simulink model "balancingControllerWithNonLinearImpedances"  (R2012b)
settings: Solver=FixedStepDiscrete  StartTime=0.0  StopTime=inf  FixedStep=Ts  RelTol=1e-3
InitFcn:
  | initBalancingControllerWithNonLinearImpedances;
values from neighbouring files (symbols this model uses):
  damping = [dampTorso,dampArms,dampArms,dampLegs,dampLegs]*0    [initBalancingControllerWithNonLinearImpedances.m]
  gainsIDMomentum = [ 0     1   1 ]    [initBalancingControllerWithNonLinearImpedances.m]
  gainsPCOM = diag([80  80 80])    [initBalancingControllerWithNonLinearImpedances.m]
  impedances = [impTorso(1,:),impArms(1,:),impArms(1,:),impLegs(1,:),impLegs(1,:)]    [initBalancingControllerWithNonLinearImpedances.m]    (also in initBalancingController_QP.m)
  impedencesSat = [100   100    2000]    [initBalancingControllerWithNonLinearImpedances.m]    (also in initBalancingController_QP.m = [100   100    1000])
  increasingRatesGainsPCOM = [ 0     0    ]    [initBalancingControllerWithNonLinearImpedances.m]
  increasingRatesImp = [impTorso(2,:),impArms(2,:),impArms(2,:),impLegs(2,:),impLegs(2,:)]    [initBalancingControllerWithNonLinearImpedances.m]    (also in initBalancingController_QP.m)
  maxCoMx_y = [ 0.1    0.05 ]    [initBalancingControllerWithNonLinearImpedances.m]
  minCoMx_y = [-0.1   -0.25 ]    [initBalancingControllerWithNonLinearImpedances.m]
  referenceParams = [0.0 0.0]    [initBalancingControllerWithNonLinearImpedances.m]    (also in initBalancingController_QP.m = [0.04 0.25])
  satGainsPCOM = 300    [initBalancingControllerWithNonLinearImpedances.m]
undefined symbols (not defined in the file or in its folder): DiscIntNeverNeededParam
libraries: WBCLibrary x22
settings Model: Creator=daniele  LastModifiedBy=daniele
settings DataIOCC: SignalLoggingSaveFormat=ModelDataLogs
settings DebuggingCC: MultiTaskDSMMsg=warning  MultiTaskCondExecSysMsg=none  FcnCallInpInsideContextMsg=EnableAllAsWarning  StrictBusMsg=None
settings SFSimCC: SimParseCustomCode=off
settings RTWCC: IncludeERTFirstTime=on
settings CodeAppCC: CustomSymbolStrType=$N$R$M_T  InternalIdentifier=Shortened
settings GRTTargetCC: CodeReplacementLibrary=None  CombineOutputUpdateFcns=off  CPPClassGenCompliant=on  GRTInterface=on

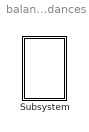
== system balancingControllerWithNonLinearImpedances ==
  Subsystem : Subsystem  mask{robotName='iCubGenova01', Ts=0.01, localName='dynamicBalancing'}
      mask prompts: robotName "robot name"; localName "module name"

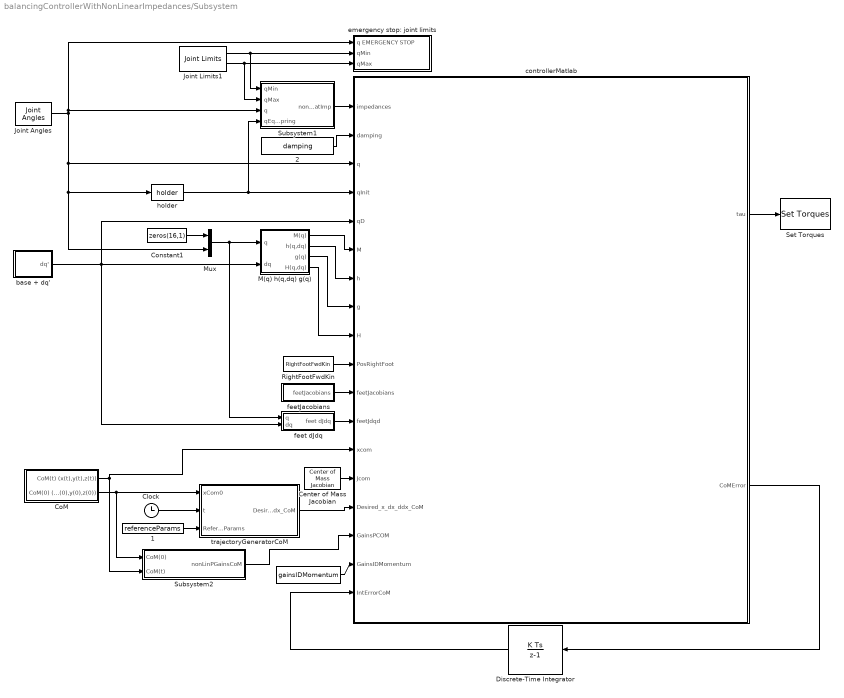
== system balancingControllerWithNonLinearImpedances/Subsystem ==
  " " : Constant  Value=gainsIDMomentum
  " 1" : Constant  Value=referenceParams
  " 2" : Constant  Value=damping
  Center of Mass Jacobian : WBCLibrary/wholeBodyModel/Jacobians/Center of Mass Jacobian  robotName=robotName  localName=localName
  Clock : Clock
  "CoM " : Subsystem
  Constant1 : Constant  Value=zeros(16,1)
  Discrete-Time Integrator : DiscreteIntegrator  InitialCondition=[0 0 0]  SampleTime=Ts  ICPrevOutput=DiscIntNeverNeededParam  ICPrevScaledInput=DiscIntNeverNeededParam
  Joint Angles : WBCLibrary/wholeBodyStates/Joint Angles  robotName=robotName  localName=localName
  Joint Limits1 : WBCLibrary/wholeBodyModel/Joint Limits  robotName=robotName  localName=localName
  M(q) h(q,dq) g(q) : Subsystem
  Mux : Mux  Inputs=2
  RightFootFwdKin : WBCLibrary/wholeBodyModel/Forward Kinematics/RightFootFwdKin  robotName=robotName  localName=localName
  Set Torques : WBCLibrary/wholeBodyActuators/Set Torques  val=6  robotName=robotName  localName=localName
  Subsystem1 : Subsystem
  Subsystem2 : Subsystem
  base + dq' : Subsystem
  controllerMatlab : MATLAB Function  TreatAsAtomicUnit=on
  emergency stop: joint limits : Subsystem
  feet dJdq : Subsystem
  feetJacobians : Subsystem
  "holder " : WBCLibrary/Utilities/holder 
  trajectoryGeneratorCoM : MATLAB Function  TreatAsAtomicUnit=on
  wires:
  trajectoryGeneratorCoM/1(Desired_x_dx_ddx_CoM) -> controllerMatlab/15(Desired_x_dx_ddx_CoM)
  Clock/1 -> trajectoryGeneratorCoM/2(t)
  "CoM "/2(CoM(0) (x(0),y(0),z(0))) -> Subsystem2/1(CoM(0)), trajectoryGeneratorCoM/1(xCom0)
  RightFootFwdKin/1 -> controllerMatlab/10(PosRightFoot)
  Discrete-Time Integrator/1 -> controllerMatlab/18(IntErrorCoM)
  Mux/1 -> M(q) h(q,dq) g(q)/1(q), feet dJdq/1(q)
  base + dq'/1(dq') -> controllerMatlab/5(qD), feet dJdq/2(dq), M(q) h(q,dq) g(q)/2(dq)
  M(q) h(q,dq) g(q)/1(M(q)) -> controllerMatlab/6(M)
  M(q) h(q,dq) g(q)/2(h(q,dq)) -> controllerMatlab/7(h)
  M(q) h(q,dq) g(q)/3(g(q)) -> controllerMatlab/8(g)
  "CoM "/1(CoM(t) (x(t),y(t),z(t))) -> Subsystem2/2(CoM(t)), controllerMatlab/13(xcom)
  M(q) h(q,dq) g(q)/4(H(q,dq)) -> controllerMatlab/9(H)
  Center of Mass Jacobian/1 -> controllerMatlab/14(Jcom)
  feetJacobians/1(feetJacobians) -> controllerMatlab/11(feetJacobians)
  feet dJdq/1(feet dJdq) -> controllerMatlab/12(feetJdqd)
  controllerMatlab/1(tau) -> Set Torques/1
  "holder "/1 -> Subsystem1/4(qEquSpring), controllerMatlab/4(qInit)
  Constant1/1 -> Mux/1
  Joint Limits1/1 -> Subsystem1/1(qMin), emergency stop: joint limits/2(qMin)
  Joint Limits1/2 -> Subsystem1/2(qMax), emergency stop: joint limits/3(qMax)
  Joint Angles/1 -> emergency stop: joint limits/1(q EMERGENCY STOP), Subsystem1/3(q), Mux/2, "holder "/1, controllerMatlab/3(q)
  Subsystem1/1(nonLinSatImp) -> controllerMatlab/1(impedances)
  controllerMatlab/2(CoMError) -> Discrete-Time Integrator/1
  " 1"/1 -> trajectoryGeneratorCoM/3(ReferenceParams)
  " "/1 -> controllerMatlab/17(GainsIDMomentum)
  Subsystem2/1(nonLinPGainsCoM) -> controllerMatlab/16(GainsPCOM)
  " 2"/1 -> controllerMatlab/2(damping)

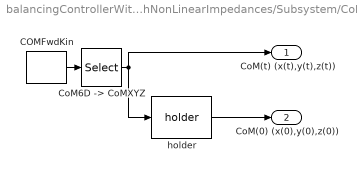
== system balancingControllerWithNonLinearImpedances/Subsystem/CoM  ==
  "COMFwdKin " : WBCLibrary/wholeBodyModel/Forward Kinematics/COMFwdKin   robotName=robotName  localName=localName
  "CoM6D -> CoMXYZ" : Selector  InputPortWidth=7  IndexOptions=Index vector (dialog)  Indices=[1 2 3]  OutputSizes=1
  "holder " : WBCLibrary/Utilities/holder 
  CoM(t) (x(t),y(t),z(t)) : Outport
  CoM(0) (x(0),y(0),z(0)) : Outport  Port=2
  wires:
  "COMFwdKin "/1 -> "CoM6D -> CoMXYZ"/1
  "CoM6D -> CoMXYZ"/1 -> "holder "/1, CoM(t) (x(t),y(t),z(t))/1
  "holder "/1 -> CoM(0) (x(0),y(0),z(0))/1

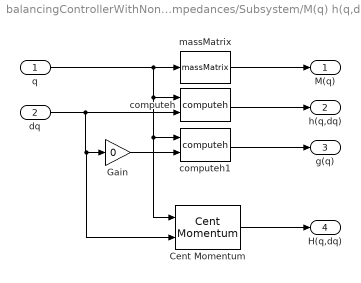
== system balancingControllerWithNonLinearImpedances/Subsystem/M(q) h(q,dq) g(q) ==
  q : Inport
  dq : Inport  Port=2
  Cent Momentum : WBCLibrary/wholeBodyModel/Dynamics/Cent Momentum  robotName=robotName  localName=localName
  Gain : Gain  Gain=0
  computeh : WBCLibrary/wholeBodyModel/Dynamics/computeh  val=7  robotname=robotName  localname=localName
  computeh1 : WBCLibrary/wholeBodyModel/Dynamics/computeh  val=7  robotname=robotName  localname=localName
  massMatrix : WBCLibrary/wholeBodyModel/Dynamics/massMatrix  val=8  robotname=robotName  localname=localName
  M(q) : Outport
  h(q,dq) : Outport  Port=2
  g(q) : Outport  Port=3
  H(q,dq) : Outport  Port=4
  wires:
  Gain/1 -> computeh1/2
  computeh1/1 -> g(q)/1
  computeh/1 -> h(q,dq)/1
  massMatrix/1 -> M(q)/1
  q/1 -> Cent Momentum/1, computeh1/1, computeh/1, massMatrix/1
  dq/1 -> Cent Momentum/2, Gain/1, computeh/2
  Cent Momentum/1 -> H(q,dq)/1

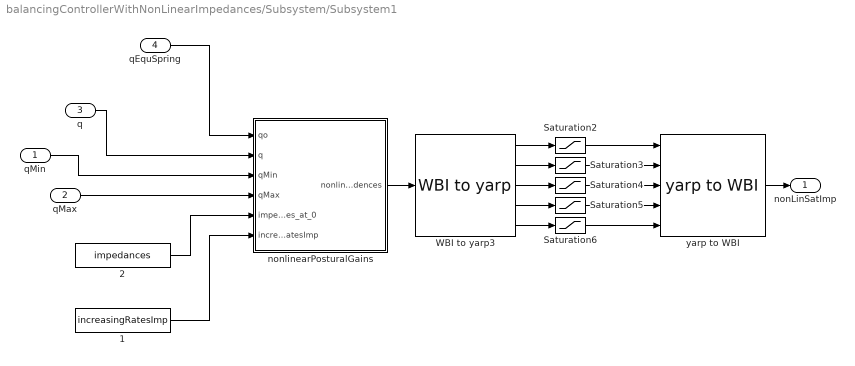
== system balancingControllerWithNonLinearImpedances/Subsystem/Subsystem1 ==
  qMin : Inport
  qMax : Inport  Port=2
  q : Inport  Port=3
  qEquSpring : Inport  Port=4
  " 1" : Constant  Value=increasingRatesImp
  " 2" : Constant  Value=impedances
  Saturation2 : Saturate  UpperLimit=impedencesSat(1)  LowerLimit=0  SampleTime=Ts
  Saturation3 : Saturate  UpperLimit=impedencesSat(2)  LowerLimit=0  SampleTime=Ts
  Saturation4 : Saturate  UpperLimit=impedencesSat(2)  LowerLimit=0  SampleTime=Ts
  Saturation5 : Saturate  UpperLimit=impedencesSat(3)  LowerLimit=0  SampleTime=Ts
  Saturation6 : Saturate  UpperLimit=impedencesSat(3)  LowerLimit=0  SampleTime=Ts
  WBI to yarp3 : WBCLibrary/Utilities/WBI to yarp
  "nonlinearPosturalGains " : MATLAB Function  TreatAsAtomicUnit=on
  yarp to WBI : WBCLibrary/Utilities/yarp to WBI
  nonLinSatImp : Outport
  wires:
  WBI to yarp3/1 -> Saturation2/1
  WBI to yarp3/2 -> Saturation3/1
  WBI to yarp3/3 -> Saturation4/1
  WBI to yarp3/4 -> Saturation5/1
  WBI to yarp3/5 -> Saturation6/1
  "nonlinearPosturalGains "/1(nonlinearImpedences) -> WBI to yarp3/1
  yarp to WBI/1 -> nonLinSatImp/1
  qEquSpring/1 -> "nonlinearPosturalGains "/1(qo)
  qMin/1 -> "nonlinearPosturalGains "/3(qMin)
  qMax/1 -> "nonlinearPosturalGains "/4(qMax)
  " 2"/1 -> "nonlinearPosturalGains "/5(impedences_at_0)
  " 1"/1 -> "nonlinearPosturalGains "/6(increasingRatesImp)
  q/1 -> "nonlinearPosturalGains "/2(q)
  Saturation6/1 -> yarp to WBI/5
  Saturation4/1 -> yarp to WBI/3
  Saturation5/1 -> yarp to WBI/4
  Saturation3/1 -> yarp to WBI/2
  Saturation2/1 -> yarp to WBI/1

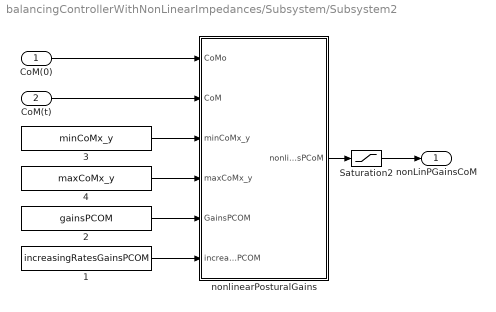
== system balancingControllerWithNonLinearImpedances/Subsystem/Subsystem2 ==
  CoM(0) : Inport
  CoM(t) : Inport  Port=2
  " 1" : Constant  Value=increasingRatesGainsPCOM
  " 2" : Constant  Value=gainsPCOM
  " 3" : Constant  Value=minCoMx_y
  " 4" : Constant  Value=maxCoMx_y
  Saturation2 : Saturate  UpperLimit=satGainsPCOM  LowerLimit=0  SampleTime=Ts
  "nonlinearPosturalGains " : MATLAB Function  TreatAsAtomicUnit=on
  nonLinPGainsCoM : Outport
  wires:
  CoM(0)/1 -> "nonlinearPosturalGains "/1(CoMo)
  " 2"/1 -> "nonlinearPosturalGains "/5(GainsPCOM)
  " 1"/1 -> "nonlinearPosturalGains "/6(increasingRatesGainsPCOM)
  CoM(t)/1 -> "nonlinearPosturalGains "/2(CoM)
  Saturation2/1 -> nonLinPGainsCoM/1
  "nonlinearPosturalGains "/1(nonlinearGainsPCoM) -> Saturation2/1
  " 4"/1 -> "nonlinearPosturalGains "/4(maxCoMx_y)
  " 3"/1 -> "nonlinearPosturalGains "/3(minCoMx_y)

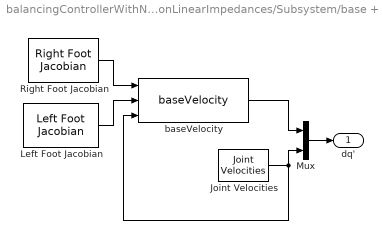
== system balancingControllerWithNonLinearImpedances/Subsystem/base + dq' ==
  Joint Velocities : WBCLibrary/wholeBodyStates/Joint Velocities  robotName=robotName  localName=localName
  Left Foot Jacobian : WBCLibrary/wholeBodyModel/Jacobians/Left Foot Jacobian  robotName=robotName  localName=localName
  Mux : Mux  Inputs=2
  Right Foot Jacobian : WBCLibrary/wholeBodyModel/Jacobians/Right Foot Jacobian  robotName=robotName  localName=localName
  baseVelocity : WBCLibrary/Utilities/baseVelocity
  dq' : Outport
  wires:
  Left Foot Jacobian/1 -> baseVelocity/2
  Right Foot Jacobian/1 -> baseVelocity/1
  baseVelocity/1 -> Mux/1
  Joint Velocities/1 -> baseVelocity/3, Mux/2
  Mux/1 -> dq'/1

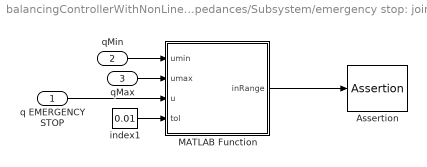
== system balancingControllerWithNonLinearImpedances/Subsystem/emergency stop: joint limits ==
  q EMERGENCY STOP : Inport
  qMin : Inport  Port=2
  qMax : Inport  Port=3
  Assertion : Assertion  Enabled=on
  MATLAB Function : MATLAB Function  TreatAsAtomicUnit=on
  index1 : Constant  Value=0.01  VectorParams1D=off
  wires:
  qMin/1 -> MATLAB Function/1(umin)
  qMax/1 -> MATLAB Function/2(umax)
  index1/1 -> MATLAB Function/4(tol)
  q EMERGENCY STOP/1 -> MATLAB Function/3(u)
  MATLAB Function/1(inRange) -> Assertion/1

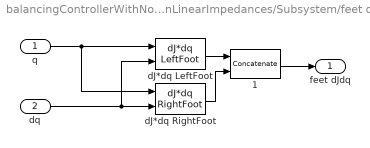
== system balancingControllerWithNonLinearImpedances/Subsystem/feet dJdq ==
  q : Inport
  dq : Inport  Port=2
  " 1" : Concatenate  Mode=Multidimensional array
  dJ*dq LeftFoot : WBCLibrary/wholeBodyModel/Dynamics/dJ*dq LeftFoot  val=9  robotName=robotName  localName=localName
  dJ*dq RightFoot : WBCLibrary/wholeBodyModel/Dynamics/dJ*dq RightFoot  val=9  robotName=robotName  localName=localName
  feet dJdq : Outport
  wires:
  dJ*dq LeftFoot/1 -> " 1"/1
  dJ*dq RightFoot/1 -> " 1"/2
  " 1"/1 -> feet dJdq/1
  q/1 -> dJ*dq RightFoot/1, dJ*dq LeftFoot/1
  dq/1 -> dJ*dq LeftFoot/2, dJ*dq RightFoot/2

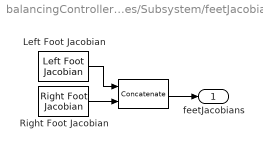
== system balancingControllerWithNonLinearImpedances/Subsystem/feetJacobians ==
  " " : Concatenate  Mode=Multidimensional array
  Left Foot Jacobian : WBCLibrary/wholeBodyModel/Jacobians/Left Foot Jacobian  robotName=robotName  localName=localName
  Right Foot Jacobian : WBCLibrary/wholeBodyModel/Jacobians/Right Foot Jacobian  robotName=robotName  localName=localName
  feetJacobians : Outport
  wires:
  Left Foot Jacobian/1 -> " "/1
  Right Foot Jacobian/1 -> " "/2
  " "/1 -> feetJacobians/1

== matlab function balancingControllerWithNonLinearImpedances/Subsystem/trajectoryGeneratorCoM ==
  data: Desired_x_dx_ddx_CoM output; xCom0 input; t input; ReferenceParams input
function Desired_x_dx_ddx_CoM = fcn(xCom0,t,ReferenceParams)
%#codegen

e3 = [0;1;0];
A = ReferenceParams(1);
f = ReferenceParams(2);

xcomDes    = xCom0 + A*sin(2*pi*f*t)*e3;
% xcomDes(1) =  xcomDes(1) + 0.01;
xDcomDes   =         A*2*pi*f*cos(2*pi*f*t)*e3;
xDDcomDes  =        -A*(2*pi*f)^2*sin(2*pi*f*t)*e3;

Desired_x_dx_ddx_CoM = [xcomDes,xDcomDes,xDDcomDes];

== matlab function balancingControllerWithNonLinearImpedances/Subsystem/controllerMatlab ==
  data: impedances input; damping input; q input; qInit input; qD input; M input; h input; g input; H input; PosRightFoot input; feetJacobians input; tau output; feetJdqd input; xcom input; Jcom input; Desired_x_dx_ddx_CoM input; GainsPCOM input; GainsIDMomentum input; CoMError output; IntErrorCoM input
function [tau,CoMError] = fcn(impedances,damping,q,qInit,qD, M, h, g, H, PosRightFoot, feetJacobians, feetJdqd, xcom,Jcom, Desired_x_dx_ddx_CoM, GainsPCOM,GainsIDMomentum, IntErrorCoM)
%#codegen
PINV_TOL = 1e-5;
gravAcc        = 9.81;

n = 25;
St    = [zeros(6,n);eye(n,n)];

m     = M(1,1);
Mb    = M(1:6,1:6);
Mbj   = M(1:6,7:end);
grav = [zeros(2,1);-m*gravAcc;zeros(3,1)];

% Definition of reference accelerations for CoM and Joints that ensure
% stabilization of desired trajectories xDcomDes and qDes 

xDcom      = Jcom(1:3,:)*qD;
xDDcomStar = Desired_x_dx_ddx_CoM(:,3) - GainsPCOM*(xcom - Desired_x_dx_ddx_CoM(:,1)) - GainsIDMomentum(1)*IntErrorCoM - GainsIDMomentum(2)*(xDcom - Desired_x_dx_ddx_CoM(:,2));

Pr =  PosRightFoot(1:3) - xcom; % Application point of the contact force on the right foot w.r.t. CoM

A  = [ eye(3),   zeros(3),eye(3), zeros(3);
      -Sf(xcom),  eye(3), Sf(Pr), eye(3) ];
pinvA = pinv(A, PINV_TOL);
  
HDotDes  = [ m*xDDcomStar ;
            -GainsIDMomentum(3)*H(4:end)]; 

Jc    =   feetJacobians;
           
JcDqD = feetJdqd;
            
desiredFeetContactForces = pinvA*(HDotDes-grav);    

JcMinv        = Jc/M;
PInv_JcMinvSt = pinv(JcMinv*St, PINV_TOL);
N0            = eye(n) - PInv_JcMinvSt*JcMinv*St;

measuredFeetContactForces = desiredFeetContactForces;

tauForDesiredFeetForces = PInv_JcMinvSt*(JcMinv*h - JcDqD - JcMinv*Jc'*measuredFeetContactForces);

tauForImpedenceBehaviour = g(7:end)-Jc(:,7:end)'*measuredFeetContactForces - impedances.*(q-qInit) - Mbj'/Mb*(h(1:6) - Jc(:,1:6)'*measuredFeetContactForces) - damping.*qD(7:end);


tau = tauForDesiredFeetForces + N0*tauForImpedenceBehaviour;

CoMError    = xcom - Desired_x_dx_ddx_CoM(:,1);

== matlab function balancingControllerWithNonLinearImpedances/Subsystem/Subsystem2/nonlinearPosturalGains  ==
  data: CoMo input; nonlinearGainsPCoM output; CoM input; minCoMx_y input; maxCoMx_y input; GainsPCOM input; increasingRatesGainsPCOM input
function nonlinearGainsPCoM = fcn(CoMo,CoM,minCoMx_y,maxCoMx_y,GainsPCOM,increasingRatesGainsPCOM)
    %#codegen

    tp =  pi./(2*(maxCoMx_y-CoMo(1:2)));
    tn = -pi./(2*(minCoMx_y-CoMo(1:2)));

    CoMTilde = CoM(1:2) - CoMo(1:2);
            
    nonlinearGainsPCoMxy      = [GainsPCOM(1,1),GainsPCOM(2,2)] + (increasingRatesGainsPCOM.*tan((tp.*stepFcn(CoMTilde) + tn.*stepFcn(-CoMTilde)).*CoMTilde).^2)' ;
    nonlinearGainsPCoM        = GainsPCOM;
    nonlinearGainsPCoM(1,1)   = nonlinearGainsPCoMxy(1);
    nonlinearGainsPCoM(2,2)   = nonlinearGainsPCoMxy(2);
end

function y = stepFcn(x) 
   %#codegen
   y = x > 0; 
end

== matlab function balancingControllerWithNonLinearImpedances/Subsystem/emergency stop: joint limits/MATLAB Function ==
  data: umin input; umax input; u input; inRange output; tol input
function inRange = checkRange(umin, umax, u, tol)
%#codegen

res = u < umin + tol | u > umax - tol;
res = sum(res);
if res==0
    inRange = 1;
else
    inRange = 0;
    u < umin + tol | u > umax - tol
end

== matlab function balancingControllerWithNonLinearImpedances/Subsystem/Subsystem1/nonlinearPosturalGains  ==
  data: qo input; nonlinearImpedences output; q input; qMin input; qMax input; impedences_at_0 input; increasingRatesImp input
function nonlinearImpedences = fcn(qo,q,qMin,qMax,impedences_at_0,increasingRatesImp)
    %#codegen

    tp =  pi./(2*(qMax-qo));
    tn = -pi./(2*(qMin-qo));

    qTilde = q - qo;
            
    nonlinearImpedences = impedences_at_0' + (increasingRatesImp.*tan((tp.*stepFcn(qTilde) + tn.*stepFcn(-qTilde)).*qTilde).^2)' ;
end

function y = stepFcn(x) 
   %#codegen
   y = x > 0; 
end
